simulink model "Quadcopter_Fix"  (R2021a)
settings: Solver=VariableStepAuto  StartTime=0.0  StopTime=50  RelTol=1e-3
values from neighbouring files (symbols this model uses):
  Ax = 0.0    (= 0)    [Quadcopter_Parameters.m]
  Ay = 0.0    (= 0)    [Quadcopter_Parameters.m]
  Az = 0.0    (= 0)    [Quadcopter_Parameters.m]
  b = 192.3208*10^(-7)    (= 1.923208e-05)    [Quadcopter_Parameters.m]
  d = 4.003*10^(-7)    (= 4.003e-07)    [Quadcopter_Parameters.m]
  g = 9.81    [Quadcopter_Parameters.m]
  Ixx = 15.67*10^(-3)    (= 0.01567)    [Quadcopter_Parameters.m]
  Iyy = 15.67*10^(-3)    (= 0.01567)    [Quadcopter_Parameters.m]
  Izz = 28.346*10^(-3)    (= 0.028346)    [Quadcopter_Parameters.m]
  Jr = 6.01*10^(-5)    (= 6.01e-05)    [Quadcopter_Parameters.m]
  l = 0.3    [Quadcopter_Parameters.m]
  m = weight/g    (= 0.815494393476)    [Quadcopter_Parameters.m]
undefined symbols (not defined in the file or in its folder): sigbuilder_block
libraries: pid_lib x6, vrlib x1
settings Model: Creator=Angga  LastModifiedBy=Angga
settings SolverCC: AlgebraicLoopSolver=TrustRegion
settings DataIOCC: ReturnWorkspaceOutputs=off
settings DebuggingCC: SFMachineParentedDataDiag=warning  ArithmeticOperatorsInVariantConditions=warning
settings SFSimCC: CustomCodeUndefinedFunction=UseInterfaceOnly

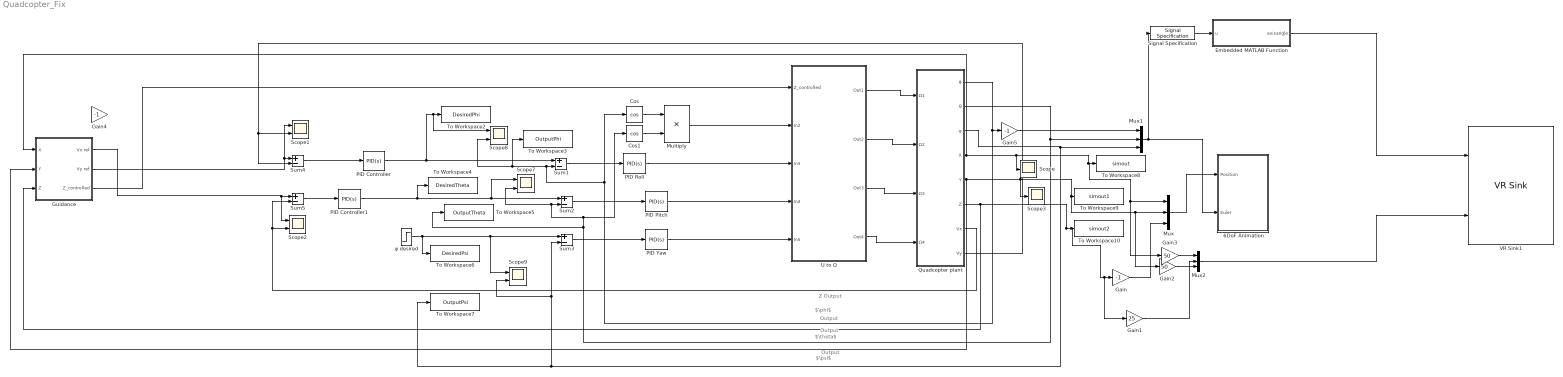
== system Quadcopter_Fix ==
  note: $\psi$
  note: $\theta$
  note: Output
  note: $\phi$
  note: Z Output
  note: Output
  note: Output
  "6DoF Animation " : Subsystem  mask{u1=[0 1 0 1 0 1], u2=0.03, u3=7, u4=[4000 0 -5000], u5=Fly alongside, u6=[-20 0 -7], u7=20, u8=off}
      mask prompts: u1 "Axes limits [xmin xmax ymin ymax zmin zmax]"; u2 "Time interval between updates:"; u3 "Size of craft displayed:"; u4 "Static object position [xp yp zp]"; u5 "Enter view:"; u6 "Position of camera [xc yc zc]"; u7 "View angle:"; u8 "Enable animation"
      mask init:
      | Config.axes = u1;
      | Config.update = u2;
      | Config.craft = u3;
      | Config.target = u4;
      | Config.camera_view = u5;
      | Config.camera_pos = u6;
      | Config.view = u7;
      | Config.Animenable = u8;
      | Config.Model = bdroot(gcb);
      mask TypeOptions u5: Fixed position | Cockpit | Fly alongside
      mask DialogControl DescGroupVar Prompt: 6DoF Animation
      mask Display:
      | port_label('input',1,'x_e','texmode','on');
      | port_label('input',2,'\phi \theta \psi','texmode','on');
      | [xp yp] = aeroimage('anim',gcbh);
      | patch(xp,yp)
  Cos : Trigonometry  Operator=cos
  Cos1 : Trigonometry  Operator=cos
  Embedded MATLAB Function : MATLAB Function  TreatAsAtomicUnit=on
  Gain : Gain  Gain=-1
  Gain1 : Gain  Gain=25
  Gain2 : Gain  Gain=50
  Gain3 : Gain  Gain=50
  Gain4 : Gain  Gain=-1
  Gain5 : Gain  Gain=-1
  Guidance : Subsystem
  Multiply : Product
  Mux : Mux  Inputs=3
  Mux1 : Mux  Inputs=3
  Mux2 : Mux  Inputs=3
  PID Controller : pid_lib/PID Controller  Controller=PID  Form=Parallel  TimeDomain=Continuous-time  UseExternalTs=off  SampleTime=-1  IntegratorMethod=Forward Euler  FilterMethod=Forward Euler  ControllerParametersSource=internal  P=-0.15  I=0  D=0  UseFilter=on  N=100  TunerSelectOption=Transfer Function Based (PID Tuner App)  InitialConditionSource=internal  InitialConditionForIntegrator=0  InitialConditionForFilter=0  DifferentiatorICPrevScaledInput=0  ExternalReset=none  TrackingMode=off  Kt=1  LimitOutput=off  SatLimitsSource=internal  UpperSaturationLimit=inf  LowerSaturationLimit=-inf  LinearizeAsGain=on  AntiWindupMode=none  Kb=1  POutMin=[]  POutMax=[]  IOutMin=[]  IOutMax=[]  DOutMin=[]  DOutMax=[]  NOutMin=[]  NOutMax=[]  SumOutMin=[]  SumOutMax=[]  SaturationOutMin=[]  SaturationOutMax=[]  PParamMin=[]  PParamMax=[]  IParamMin=[]  IParamMax=[]  DParamMin=[]  DParamMax=[]  NParamMin=[]  NParamMax=[]  KbParamMin=[]  KbParamMax=[]  KtParamMin=[]  KtParamMax=[]  KbOutMin=[]  KbOutMax=[]  KtOutMin=[]  KtOutMax=[]  IntegratorOutMin=[]  IntegratorOutMax=[]  FilterOutMin=[]  FilterOutMax=[]  SumI1OutMin=[]  SumI1OutMax=[]  SumI2OutMin=[]  SumI2OutMax=[]  SumI3OutMin=[]  SumI3OutMax=[]  SumI4OutMin=[]  SumI4OutMax=[]  SumDOutMin=[]  SumDOutMax=[]  DifferentiatorOutMin=[]  DifferentiatorOutMax=[]  FilterDiffOutCoefMin=[]  FilterDiffOutCoefMax=[]  ReciprocalOutMin=[]  ReciprocalOutMax=[]  SumDenOutMin=[]  SumDenOutMax=[]  SumNumOutMin=[]  SumNumOutMax=[]  DivideOutMin=[]  DivideOutMax=[]  UdiffTsProdOutMin=[]  UdiffTsProdOutMax=[]  NTsProdOutMin=[]  NTsProdOutMax=[]  UintegralTsProdOutMin=[]  UintegralTsProdOutMax=[]  UngainTsProdOutMin=[]  UngainTsProdOutMax=[]  IntegratorContinuousStateAttributes=''  IntegratorStateMustResolveToSignalObject=off  IntegratorRTWStateStorageClass=Auto  FilterContinuousStateAttributes=''  FilterStateMustResolveToSignalObject=off  FilterRTWStateStorageClass=Auto  ParallelPVariant=InternalParameters  IdealPVariant=Disabled  IVariant=InternalParameters  DVariant=InternalParameters  IntegratorVariant=Continuous  SatVariant=Disabled  AWVariant=Passthrough  PCopyVariant=Disabled  TRVariant=Disabled  FdbkBlocksVariant=Forward  IdealPFdbkVariant=Disabled  SatFdbkVariant=Disabled  DerivativeFilterVariant=ContFilter  NVariant=InternalParameters  NCopyVariant=Disabled  FilterICVariant=InternalICsFilter  IntegratorICVariant=InternalICs  ExternalResetVariant=Disabled  TRSumVariant=Passthrough  SumFdbkVariant=Disabled  SumVariant=Sum_PID  TsampFilterVariant=InternalTs  TsampNgainVariant=Passthrough  TsampIntegralVariant=Passthrough  ExternalSaturationOutDataTypeStr=Inherit: Same as second input
  PID Controller1 : pid_lib/PID Controller  Controller=PID  Form=Parallel  TimeDomain=Continuous-time  UseExternalTs=off  SampleTime=-1  IntegratorMethod=Forward Euler  FilterMethod=Forward Euler  ControllerParametersSource=internal  P=-0.2  I=0  D=0  UseFilter=on  N=100  TunerSelectOption=Transfer Function Based (PID Tuner App)  InitialConditionSource=internal  InitialConditionForIntegrator=0  InitialConditionForFilter=0  DifferentiatorICPrevScaledInput=0  ExternalReset=none  TrackingMode=off  Kt=1  LimitOutput=off  SatLimitsSource=internal  UpperSaturationLimit=inf  LowerSaturationLimit=-inf  LinearizeAsGain=on  AntiWindupMode=none  Kb=1  POutMin=[]  POutMax=[]  IOutMin=[]  IOutMax=[]  DOutMin=[]  DOutMax=[]  NOutMin=[]  NOutMax=[]  SumOutMin=[]  SumOutMax=[]  SaturationOutMin=[]  SaturationOutMax=[]  PParamMin=[]  PParamMax=[]  IParamMin=[]  IParamMax=[]  DParamMin=[]  DParamMax=[]  NParamMin=[]  NParamMax=[]  KbParamMin=[]  KbParamMax=[]  KtParamMin=[]  KtParamMax=[]  KbOutMin=[]  KbOutMax=[]  KtOutMin=[]  KtOutMax=[]  IntegratorOutMin=[]  IntegratorOutMax=[]  FilterOutMin=[]  FilterOutMax=[]  SumI1OutMin=[]  SumI1OutMax=[]  SumI2OutMin=[]  SumI2OutMax=[]  SumI3OutMin=[]  SumI3OutMax=[]  SumI4OutMin=[]  SumI4OutMax=[]  SumDOutMin=[]  SumDOutMax=[]  DifferentiatorOutMin=[]  DifferentiatorOutMax=[]  FilterDiffOutCoefMin=[]  FilterDiffOutCoefMax=[]  ReciprocalOutMin=[]  ReciprocalOutMax=[]  SumDenOutMin=[]  SumDenOutMax=[]  SumNumOutMin=[]  SumNumOutMax=[]  DivideOutMin=[]  DivideOutMax=[]  UdiffTsProdOutMin=[]  UdiffTsProdOutMax=[]  NTsProdOutMin=[]  NTsProdOutMax=[]  UintegralTsProdOutMin=[]  UintegralTsProdOutMax=[]  UngainTsProdOutMin=[]  UngainTsProdOutMax=[]  IntegratorContinuousStateAttributes=''  IntegratorStateMustResolveToSignalObject=off  IntegratorRTWStateStorageClass=Auto  FilterContinuousStateAttributes=''  FilterStateMustResolveToSignalObject=off  FilterRTWStateStorageClass=Auto  ParallelPVariant=InternalParameters  IdealPVariant=Disabled  IVariant=InternalParameters  DVariant=InternalParameters  IntegratorVariant=Continuous  SatVariant=Disabled  AWVariant=Passthrough  PCopyVariant=Disabled  TRVariant=Disabled  FdbkBlocksVariant=Forward  IdealPFdbkVariant=Disabled  SatFdbkVariant=Disabled  DerivativeFilterVariant=ContFilter  NVariant=InternalParameters  NCopyVariant=Disabled  FilterICVariant=InternalICsFilter  IntegratorICVariant=InternalICs  ExternalResetVariant=Disabled  TRSumVariant=Passthrough  SumFdbkVariant=Disabled  SumVariant=Sum_PID  TsampFilterVariant=InternalTs  TsampNgainVariant=Passthrough  TsampIntegralVariant=Passthrough  ExternalSaturationOutDataTypeStr=Inherit: Same as second input
  PID Pitch : pid_lib/PID Controller  Controller=PID  Form=Parallel  TimeDomain=Continuous-time  UseExternalTs=off  SampleTime=-1  IntegratorMethod=Forward Euler  FilterMethod=Forward Euler  ControllerParametersSource=internal  P=0.05  I=0  D=0.05  UseFilter=on  N=100  TunerSelectOption=Transfer Function Based (PID Tuner App)  InitialConditionSource=internal  InitialConditionForIntegrator=0  InitialConditionForFilter=0  DifferentiatorICPrevScaledInput=0  ExternalReset=none  TrackingMode=off  Kt=1  LimitOutput=off  SatLimitsSource=internal  UpperSaturationLimit=inf  LowerSaturationLimit=-inf  LinearizeAsGain=on  AntiWindupMode=none  Kb=1  POutMin=[]  POutMax=[]  IOutMin=[]  IOutMax=[]  DOutMin=[]  DOutMax=[]  NOutMin=[]  NOutMax=[]  SumOutMin=[]  SumOutMax=[]  SaturationOutMin=[]  SaturationOutMax=[]  PParamMin=[]  PParamMax=[]  IParamMin=[]  IParamMax=[]  DParamMin=[]  DParamMax=[]  NParamMin=[]  NParamMax=[]  KbParamMin=[]  KbParamMax=[]  KtParamMin=[]  KtParamMax=[]  KbOutMin=[]  KbOutMax=[]  KtOutMin=[]  KtOutMax=[]  IntegratorOutMin=[]  IntegratorOutMax=[]  FilterOutMin=[]  FilterOutMax=[]  SumI1OutMin=[]  SumI1OutMax=[]  SumI2OutMin=[]  SumI2OutMax=[]  SumI3OutMin=[]  SumI3OutMax=[]  SumI4OutMin=[]  SumI4OutMax=[]  SumDOutMin=[]  SumDOutMax=[]  DifferentiatorOutMin=[]  DifferentiatorOutMax=[]  FilterDiffOutCoefMin=[]  FilterDiffOutCoefMax=[]  ReciprocalOutMin=[]  ReciprocalOutMax=[]  SumDenOutMin=[]  SumDenOutMax=[]  SumNumOutMin=[]  SumNumOutMax=[]  DivideOutMin=[]  DivideOutMax=[]  UdiffTsProdOutMin=[]  UdiffTsProdOutMax=[]  NTsProdOutMin=[]  NTsProdOutMax=[]  UintegralTsProdOutMin=[]  UintegralTsProdOutMax=[]  UngainTsProdOutMin=[]  UngainTsProdOutMax=[]  IntegratorContinuousStateAttributes=''  IntegratorStateMustResolveToSignalObject=off  IntegratorRTWStateStorageClass=Auto  FilterContinuousStateAttributes=''  FilterStateMustResolveToSignalObject=off  FilterRTWStateStorageClass=Auto  ParallelPVariant=InternalParameters  IdealPVariant=Disabled  IVariant=InternalParameters  DVariant=InternalParameters  IntegratorVariant=Continuous  SatVariant=Disabled  AWVariant=Passthrough  PCopyVariant=Disabled  TRVariant=Disabled  FdbkBlocksVariant=Forward  IdealPFdbkVariant=Disabled  SatFdbkVariant=Disabled  DerivativeFilterVariant=ContFilter  NVariant=InternalParameters  NCopyVariant=Disabled  FilterICVariant=InternalICsFilter  IntegratorICVariant=InternalICs  ExternalResetVariant=Disabled  TRSumVariant=Passthrough  SumFdbkVariant=Disabled  SumVariant=Sum_PID  TsampFilterVariant=InternalTs  TsampNgainVariant=Passthrough  TsampIntegralVariant=Passthrough  ExternalSaturationOutDataTypeStr=Inherit: Same as second input
  PID Roll : pid_lib/PID Controller  Controller=PID  Form=Parallel  TimeDomain=Continuous-time  UseExternalTs=off  SampleTime=-1  IntegratorMethod=Forward Euler  FilterMethod=Forward Euler  ControllerParametersSource=internal  P=0.05  I=0  D=0.05  UseFilter=on  N=100  TunerSelectOption=Transfer Function Based (PID Tuner App)  InitialConditionSource=internal  InitialConditionForIntegrator=0  InitialConditionForFilter=0  DifferentiatorICPrevScaledInput=0  ExternalReset=none  TrackingMode=off  Kt=1  LimitOutput=off  SatLimitsSource=internal  UpperSaturationLimit=inf  LowerSaturationLimit=-inf  LinearizeAsGain=on  AntiWindupMode=none  Kb=1  POutMin=[]  POutMax=[]  IOutMin=[]  IOutMax=[]  DOutMin=[]  DOutMax=[]  NOutMin=[]  NOutMax=[]  SumOutMin=[]  SumOutMax=[]  SaturationOutMin=[]  SaturationOutMax=[]  PParamMin=[]  PParamMax=[]  IParamMin=[]  IParamMax=[]  DParamMin=[]  DParamMax=[]  NParamMin=[]  NParamMax=[]  KbParamMin=[]  KbParamMax=[]  KtParamMin=[]  KtParamMax=[]  KbOutMin=[]  KbOutMax=[]  KtOutMin=[]  KtOutMax=[]  IntegratorOutMin=[]  IntegratorOutMax=[]  FilterOutMin=[]  FilterOutMax=[]  SumI1OutMin=[]  SumI1OutMax=[]  SumI2OutMin=[]  SumI2OutMax=[]  SumI3OutMin=[]  SumI3OutMax=[]  SumI4OutMin=[]  SumI4OutMax=[]  SumDOutMin=[]  SumDOutMax=[]  DifferentiatorOutMin=[]  DifferentiatorOutMax=[]  FilterDiffOutCoefMin=[]  FilterDiffOutCoefMax=[]  ReciprocalOutMin=[]  ReciprocalOutMax=[]  SumDenOutMin=[]  SumDenOutMax=[]  SumNumOutMin=[]  SumNumOutMax=[]  DivideOutMin=[]  DivideOutMax=[]  UdiffTsProdOutMin=[]  UdiffTsProdOutMax=[]  NTsProdOutMin=[]  NTsProdOutMax=[]  UintegralTsProdOutMin=[]  UintegralTsProdOutMax=[]  UngainTsProdOutMin=[]  UngainTsProdOutMax=[]  IntegratorContinuousStateAttributes=''  IntegratorStateMustResolveToSignalObject=off  IntegratorRTWStateStorageClass=Auto  FilterContinuousStateAttributes=''  FilterStateMustResolveToSignalObject=off  FilterRTWStateStorageClass=Auto  ParallelPVariant=InternalParameters  IdealPVariant=Disabled  IVariant=InternalParameters  DVariant=InternalParameters  IntegratorVariant=Continuous  SatVariant=Disabled  AWVariant=Passthrough  PCopyVariant=Disabled  TRVariant=Disabled  FdbkBlocksVariant=Forward  IdealPFdbkVariant=Disabled  SatFdbkVariant=Disabled  DerivativeFilterVariant=ContFilter  NVariant=InternalParameters  NCopyVariant=Disabled  FilterICVariant=InternalICsFilter  IntegratorICVariant=InternalICs  ExternalResetVariant=Disabled  TRSumVariant=Passthrough  SumFdbkVariant=Disabled  SumVariant=Sum_PID  TsampFilterVariant=InternalTs  TsampNgainVariant=Passthrough  TsampIntegralVariant=Passthrough  ExternalSaturationOutDataTypeStr=Inherit: Same as second input
  PID Yaw : pid_lib/PID Controller  Controller=PID  Form=Parallel  TimeDomain=Continuous-time  UseExternalTs=off  SampleTime=-1  IntegratorMethod=Forward Euler  FilterMethod=Forward Euler  ControllerParametersSource=internal  P=0.05  I=0  D=0.05  UseFilter=on  N=100  TunerSelectOption=Transfer Function Based (PID Tuner App)  InitialConditionSource=internal  InitialConditionForIntegrator=0  InitialConditionForFilter=0  DifferentiatorICPrevScaledInput=0  ExternalReset=none  TrackingMode=off  Kt=1  LimitOutput=off  SatLimitsSource=internal  UpperSaturationLimit=inf  LowerSaturationLimit=-inf  LinearizeAsGain=on  AntiWindupMode=none  Kb=1  POutMin=[]  POutMax=[]  IOutMin=[]  IOutMax=[]  DOutMin=[]  DOutMax=[]  NOutMin=[]  NOutMax=[]  SumOutMin=[]  SumOutMax=[]  SaturationOutMin=[]  SaturationOutMax=[]  PParamMin=[]  PParamMax=[]  IParamMin=[]  IParamMax=[]  DParamMin=[]  DParamMax=[]  NParamMin=[]  NParamMax=[]  KbParamMin=[]  KbParamMax=[]  KtParamMin=[]  KtParamMax=[]  KbOutMin=[]  KbOutMax=[]  KtOutMin=[]  KtOutMax=[]  IntegratorOutMin=[]  IntegratorOutMax=[]  FilterOutMin=[]  FilterOutMax=[]  SumI1OutMin=[]  SumI1OutMax=[]  SumI2OutMin=[]  SumI2OutMax=[]  SumI3OutMin=[]  SumI3OutMax=[]  SumI4OutMin=[]  SumI4OutMax=[]  SumDOutMin=[]  SumDOutMax=[]  DifferentiatorOutMin=[]  DifferentiatorOutMax=[]  FilterDiffOutCoefMin=[]  FilterDiffOutCoefMax=[]  ReciprocalOutMin=[]  ReciprocalOutMax=[]  SumDenOutMin=[]  SumDenOutMax=[]  SumNumOutMin=[]  SumNumOutMax=[]  DivideOutMin=[]  DivideOutMax=[]  UdiffTsProdOutMin=[]  UdiffTsProdOutMax=[]  NTsProdOutMin=[]  NTsProdOutMax=[]  UintegralTsProdOutMin=[]  UintegralTsProdOutMax=[]  UngainTsProdOutMin=[]  UngainTsProdOutMax=[]  IntegratorContinuousStateAttributes=''  IntegratorStateMustResolveToSignalObject=off  IntegratorRTWStateStorageClass=Auto  FilterContinuousStateAttributes=''  FilterStateMustResolveToSignalObject=off  FilterRTWStateStorageClass=Auto  ParallelPVariant=InternalParameters  IdealPVariant=Disabled  IVariant=InternalParameters  DVariant=InternalParameters  IntegratorVariant=Continuous  SatVariant=Disabled  AWVariant=Passthrough  PCopyVariant=Disabled  TRVariant=Disabled  FdbkBlocksVariant=Forward  IdealPFdbkVariant=Disabled  SatFdbkVariant=Disabled  DerivativeFilterVariant=ContFilter  NVariant=InternalParameters  NCopyVariant=Disabled  FilterICVariant=InternalICsFilter  IntegratorICVariant=InternalICs  ExternalResetVariant=Disabled  TRSumVariant=Passthrough  SumFdbkVariant=Disabled  SumVariant=Sum_PID  TsampFilterVariant=InternalTs  TsampNgainVariant=Passthrough  TsampIntegralVariant=Passthrough  ExternalSaturationOutDataTypeStr=Inherit: Same as second input
  Quadcopter plant : Subsystem
  Scope : Scope
  Scope{1..2,7..9} (5 alike) : Scope  NumInputPorts=2
  Scope3 : Scope
  Signal Specification : SignalSpecification  Dimensions=3
  Sum{1..5} (5 alike) : Sum  Inputs=+-
  To Workspace10 : ToWorkspace  VariableName=simout2  SampleTime=-1
  To Workspace2 : ToWorkspace  VariableName=DesiredPhi  SampleTime=-1
  To Workspace3 : ToWorkspace  VariableName=OutputPhi  SampleTime=-1
  To Workspace4 : ToWorkspace  VariableName=DesiredTheta  SampleTime=-1
  To Workspace5 : ToWorkspace  VariableName=OutputTheta  SampleTime=-1
  To Workspace6 : ToWorkspace  VariableName=DesiredPsi  SampleTime=-1
  To Workspace7 : ToWorkspace  VariableName=OutputPsi  SampleTime=-1
  To Workspace8 : ToWorkspace  VariableName=simout  SampleTime=-1
  To Workspace9 : ToWorkspace  VariableName=simout1  SampleTime=-1
  U to Ω : Subsystem
  VR Sink1 : vrlib/VR Sink  InstantiateOnLoad=on  SampleTime=0.05  ViewEnable=on  RemoteChange=off  RemoteView=on  FieldsWritten=STLB_Transform.rotation.4.1.1.double#STLB_Transform.translation.3.1.1.double  WorldFileName=Quadcopter.x3d  AutoView=on  VideoDimensions=[]  AllowVariableSize=off
  ψ desired : Step  After=0  SampleTime=0
  wires:
  Quadcopter plant/3(ψ) -> Sum3/2, Scope9/2, To Workspace7/1, Mux1/3
  Quadcopter plant/4(X) -> Guidance/1(X), Scope/1, Gain3/1, Mux/1, To Workspace8/1
  Quadcopter plant/1(ϕ) -> To Workspace3/1, Scope8/2, Sum1/2, Cos/1, Gain5/1
  Quadcopter plant/2(θ) -> Cos1/1, Scope7/2, Sum2/2, To Workspace5/1, Mux1/2
  Quadcopter plant/6(Z) -> Guidance/3(Z), Gain1/1, Gain/1, To Workspace10/1
  Cos/1 -> Multiply/1
  Cos1/1 -> Multiply/2
  Sum1/1 -> PID Roll/1
  Sum2/1 -> PID Pitch/1
  ψ desired/1 -> To Workspace6/1, Scope9/1, Sum3/1
  Sum3/1 -> PID Yaw/1
  Mux/1 -> "6DoF Animation "/1(Position)
  Mux1/1 -> Signal Specification/1, "6DoF Animation "/2(Euler)
  Gain/1 -> Mux/3
  Multiply/1 -> U to Ω/2(In2)
  PID Roll/1 -> U to Ω/3(In3)
  PID Pitch/1 -> U to Ω/4(In4)
  PID Yaw/1 -> U to Ω/5(In5)
  U to Ω/1(Out1) -> Quadcopter plant/1(Ω1)
  U to Ω/2(Out2) -> Quadcopter plant/2(Ω2)
  U to Ω/3(Out3) -> Quadcopter plant/3(Ω3)
  U to Ω/4(Out4) -> Quadcopter plant/4(Ω4)
  Signal Specification/1 -> Embedded MATLAB Function/1(u)
  Embedded MATLAB Function/1(axisangle) -> VR Sink1/1
  Mux2/1 -> VR Sink1/2
  Gain1/1 -> Mux2/2
  PID Controller/1 -> Sum1/1, Scope8/1, To Workspace2/1
  PID Controller1/1 -> To Workspace4/1, Sum2/1, Scope7/1
  Quadcopter plant/8(Vy) -> Scope1/2, Sum4/2
  Sum4/1 -> PID Controller/1
  Quadcopter plant/7(Vx) -> Sum5/2, Scope2/2
  Sum5/1 -> PID Controller1/1
  Guidance/3(Z_controlled) -> U to Ω/1(Z_controlled)
  Guidance/2(Vy ref) -> Scope1/1, Sum4/1
  Guidance/1(Vx ref) -> Scope2/1, Sum5/1
  Gain2/1 -> Mux2/3
  Gain3/1 -> Mux2/1
  Quadcopter plant/5(Y) -> Scope3/1, Gain2/1, Mux/2, To Workspace9/1, Guidance/2(Y)
  Gain5/1 -> Mux1/1

== system Quadcopter_Fix/6DoF Animation  ==
  Position : Inport
  Euler : Inport  Port=2
  Animation S-Function : S-Function  FunctionName=sixdofanim  Parameters=Config  SFunctionDeploymentMode=off  EnableBusSupport=off
  Mux3 : Mux  Inputs=2
  wires:
  Mux3/1 -> Animation S-Function/1
  Position/1 -> Mux3/1
  Euler/1 -> Mux3/2

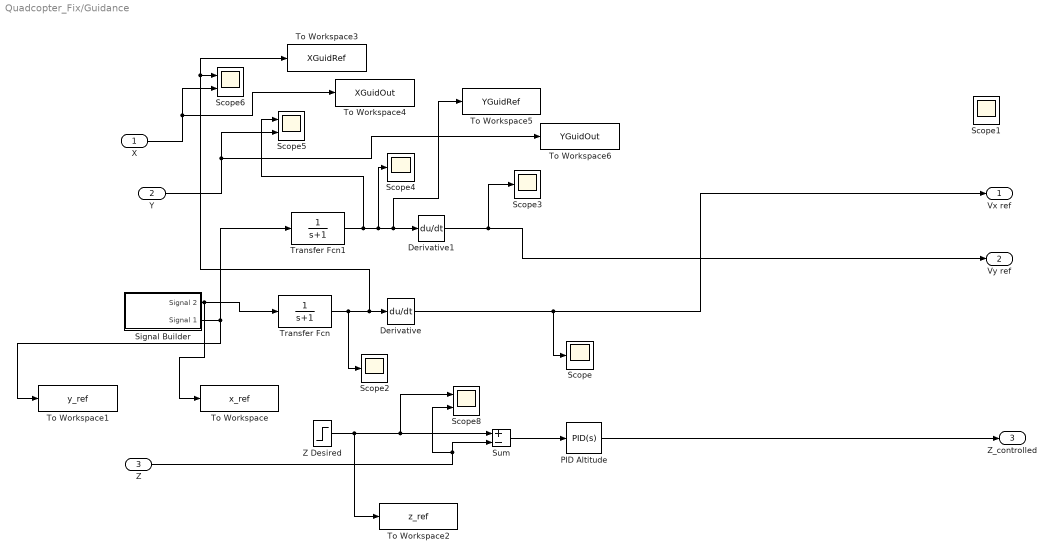
== system Quadcopter_Fix/Guidance ==
  X : Inport
  Y : Inport  Port=2
  Z : Inport  Port=3
  Derivative : Derivative
  Derivative1 : Derivative
  PID Altitude : pid_lib/PID Controller  Controller=PID  Form=Parallel  TimeDomain=Continuous-time  UseExternalTs=off  SampleTime=-1  IntegratorMethod=Forward Euler  FilterMethod=Forward Euler  ControllerParametersSource=internal  P=6  I=3  D=3  UseFilter=on  N=100  TunerSelectOption=Transfer Function Based (PID Tuner App)  InitialConditionSource=internal  InitialConditionForIntegrator=0  InitialConditionForFilter=0  DifferentiatorICPrevScaledInput=0  ExternalReset=none  TrackingMode=off  Kt=1  LimitOutput=off  SatLimitsSource=internal  UpperSaturationLimit=inf  LowerSaturationLimit=-inf  LinearizeAsGain=on  AntiWindupMode=none  Kb=1  POutMin=[]  POutMax=[]  IOutMin=[]  IOutMax=[]  DOutMin=[]  DOutMax=[]  NOutMin=[]  NOutMax=[]  SumOutMin=[]  SumOutMax=[]  SaturationOutMin=[]  SaturationOutMax=[]  PParamMin=[]  PParamMax=[]  IParamMin=[]  IParamMax=[]  DParamMin=[]  DParamMax=[]  NParamMin=[]  NParamMax=[]  KbParamMin=[]  KbParamMax=[]  KtParamMin=[]  KtParamMax=[]  KbOutMin=[]  KbOutMax=[]  KtOutMin=[]  KtOutMax=[]  IntegratorOutMin=[]  IntegratorOutMax=[]  FilterOutMin=[]  FilterOutMax=[]  SumI1OutMin=[]  SumI1OutMax=[]  SumI2OutMin=[]  SumI2OutMax=[]  SumI3OutMin=[]  SumI3OutMax=[]  SumI4OutMin=[]  SumI4OutMax=[]  SumDOutMin=[]  SumDOutMax=[]  DifferentiatorOutMin=[]  DifferentiatorOutMax=[]  FilterDiffOutCoefMin=[]  FilterDiffOutCoefMax=[]  ReciprocalOutMin=[]  ReciprocalOutMax=[]  SumDenOutMin=[]  SumDenOutMax=[]  SumNumOutMin=[]  SumNumOutMax=[]  DivideOutMin=[]  DivideOutMax=[]  UdiffTsProdOutMin=[]  UdiffTsProdOutMax=[]  NTsProdOutMin=[]  NTsProdOutMax=[]  UintegralTsProdOutMin=[]  UintegralTsProdOutMax=[]  UngainTsProdOutMin=[]  UngainTsProdOutMax=[]  IntegratorContinuousStateAttributes=''  IntegratorStateMustResolveToSignalObject=off  IntegratorRTWStateStorageClass=Auto  FilterContinuousStateAttributes=''  FilterStateMustResolveToSignalObject=off  FilterRTWStateStorageClass=Auto  ParallelPVariant=InternalParameters  IdealPVariant=Disabled  IVariant=InternalParameters  DVariant=InternalParameters  IntegratorVariant=Continuous  SatVariant=Disabled  AWVariant=Passthrough  PCopyVariant=Disabled  TRVariant=Disabled  FdbkBlocksVariant=Forward  IdealPFdbkVariant=Disabled  SatFdbkVariant=Disabled  DerivativeFilterVariant=ContFilter  NVariant=InternalParameters  NCopyVariant=Disabled  FilterICVariant=InternalICsFilter  IntegratorICVariant=InternalICs  ExternalResetVariant=Disabled  TRSumVariant=Passthrough  SumFdbkVariant=Disabled  SumVariant=Sum_PID  TsampFilterVariant=InternalTs  TsampNgainVariant=Passthrough  TsampIntegralVariant=Passthrough  ExternalSaturationOutDataTypeStr=Inherit: Same as second input
  Scope{,1..4} (5 alike) : Scope
  Scope5 : Scope  NumInputPorts=2
  Scope6 : Scope  NumInputPorts=2
  Scope8 : Scope  NumInputPorts=2
  Signal Builder : Subsystem  Tag=STV Subsys  LoadFcn=sigbuilder_block('load');  StartFcn=sigbuilder_block('start');  StopFcn=sigbuilder_block('stop');  ClipboardFcn=sigbuilder_block('clipboard');  mask(Sigbuilder block){tuvar=[0:10]}
      mask help: Simulink:masks:SigbuilderBlock_MD
      mask init:
      | if ~strcmp(get_param(bdroot(gcbh),'SimulationStatus'),'stopped') tuvar = sigbuilder_block('maskInit'); end
      settings: CopyFcn=sigbuilder_block('copy');  DeleteFcn=sigbuilder_block('delete');  ModelCloseFcn=sigbuilder_block('modelClose');  PreSaveFcn=sigbuilder_block('preSave');  PauseFcn=sigbuilder_block('pause');  ContinueFcn=sigbuilder_block('continue');  NameChangeFcn=sigbuilder_block('namechange');  OpenFcn=sigbuilder_block('open',[5.5 -8 949 380.5 ]);  CloseFcn=sigbuilder_block('close');
      mask Display: plot(0, 0, 100, 100,[2, 2, 32, 32, 2], [68, 8, 8, 68, 68],[32, 2], [38, 38], [32, 19, 2],[53, 60, 44], [32, 17, 17, 2],[16, 16, 31, 31]);txt = getActiveGroup(gcbh);text(2, 100, txt,'verticalAlignment', 'top');
  Sum : Sum  Inputs=+-
  To Workspace : ToWorkspace  VariableName=x_ref  SampleTime=-1
  To Workspace1 : ToWorkspace  VariableName=y_ref  SampleTime=-1
  To Workspace2 : ToWorkspace  VariableName=z_ref  SampleTime=-1
  To Workspace3 : ToWorkspace  VariableName=XGuidRef  SampleTime=-1
  To Workspace4 : ToWorkspace  VariableName=XGuidOut  SampleTime=-1
  To Workspace5 : ToWorkspace  VariableName=YGuidRef  SampleTime=-1
  To Workspace6 : ToWorkspace  VariableName=YGuidOut  SampleTime=-1
  Transfer Fcn : TransferFcn  Denominator=[1 1]
  Transfer Fcn1 : TransferFcn  Denominator=[1 1]
  Z Desired : Step  After=5  SampleTime=0
  Vx ref : Outport
  Vy ref : Outport  Port=2
  Z_controlled : Outport  Port=3
  wires:
  Sum/1 -> PID Altitude/1
  Z Desired/1 -> To Workspace2/1, Scope8/1, Sum/1
  Z/1 -> Scope8/2, Sum/2
  PID Altitude/1 -> Z_controlled/1
  Signal Builder/1(Signal 2) -> To Workspace/1, Transfer Fcn/1
  Transfer Fcn/1 -> Scope2/1, To Workspace3/1, Scope6/1, Derivative/1
  Derivative/1 -> Scope/1, Vx ref/1
  Signal Builder/2(Signal 1) -> To Workspace1/1, Transfer Fcn1/1
  Transfer Fcn1/1 -> Scope5/1, Scope4/1, To Workspace5/1, Derivative1/1
  Derivative1/1 -> Scope3/1, Vy ref/1
  Y/1 -> To Workspace6/1, Scope5/2
  X/1 -> To Workspace4/1, Scope6/2

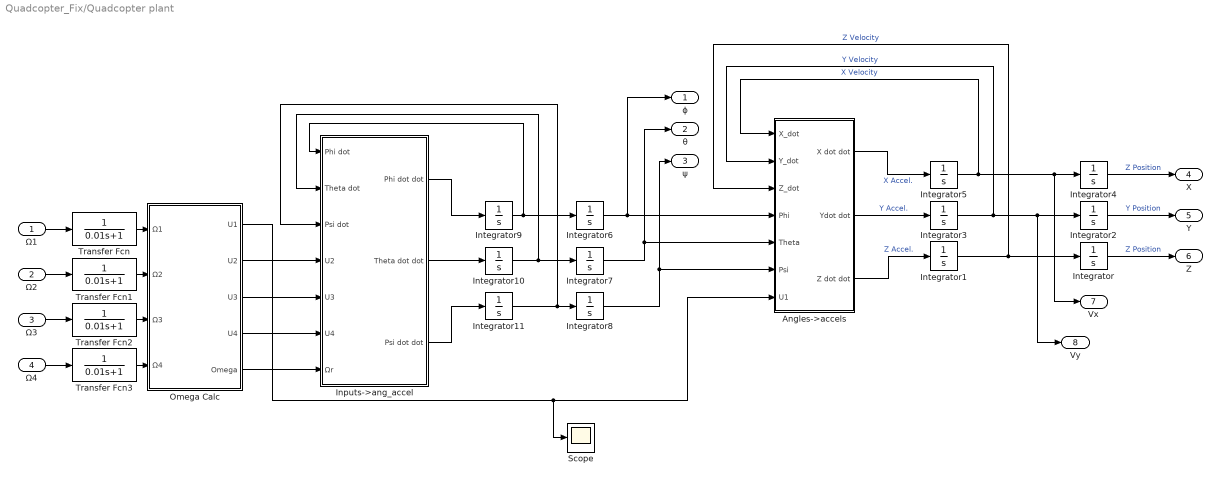
== system Quadcopter_Fix/Quadcopter plant ==
  Ω1 : Inport
  Ω2 : Inport  Port=2
  Ω3 : Inport  Port=3
  Ω4 : Inport  Port=4
  Angles->accels : Subsystem
  Inputs->ang_accel : Subsystem
  Integrator : Integrator  LimitOutput=on  LowerSaturationLimit=0
  Integrator{1..5,8..9} (7 alike) : Integrator
  Integrator10 : Integrator  UpperSaturationLimit=10000  LowerSaturationLimit=-10000
  Integrator11 : Integrator  UpperSaturationLimit=10000  LowerSaturationLimit=-10000
  Integrator6 : Integrator  WrapState=on  WrappedStateUpperValue=pi/2  WrappedStateLowerValue=-pi/2
  Integrator7 : Integrator  WrapState=on  WrappedStateUpperValue=pi/3  WrappedStateLowerValue=-pi/3
  Omega Calc : Subsystem
  Scope : Scope
  Transfer Fcn{,1..3} (4 alike) : TransferFcn  Denominator=[0.01 1]
  ϕ : Outport  VectorParamsAs1DForOutWhenUnconnected=off
  θ : Outport  Port=2  VectorParamsAs1DForOutWhenUnconnected=off
  ψ : Outport  Port=3  VectorParamsAs1DForOutWhenUnconnected=off
  X : Outport  Port=4  VectorParamsAs1DForOutWhenUnconnected=off
  Y : Outport  Port=5  VectorParamsAs1DForOutWhenUnconnected=off
  Z : Outport  Port=6  VectorParamsAs1DForOutWhenUnconnected=off
  Vx : Outport  Port=7  VectorParamsAs1DForOutWhenUnconnected=off
  Vy : Outport  Port=8  VectorParamsAs1DForOutWhenUnconnected=off
  wires:
  Integrator1/1 -> Angles->accels/3(Z_dot), Integrator/1  "Z Velocity"
  Integrator2/1 -> Y/1  "Y Position"
  Integrator3/1 -> Angles->accels/2(Y_dot), Vy/1, Integrator2/1  "Y Velocity"
  Angles->accels/2(Ydot dot) -> Integrator3/1  "Y Accel."
  Angles->accels/3(Z dot dot) -> Integrator1/1  "Z Accel."
  Integrator8/1 -> Angles->accels/6(Psi), ψ/1
  Integrator7/1 -> Angles->accels/5(Theta), θ/1
  Integrator6/1 -> Angles->accels/4(Phi), ϕ/1
  Integrator11/1 -> Inputs->ang_accel/3(Psi dot), Integrator8/1
  Integrator10/1 -> Inputs->ang_accel/2(Theta dot), Integrator7/1
  Integrator9/1 -> Inputs->ang_accel/1(Phi dot), Integrator6/1
  Inputs->ang_accel/2(Theta dot dot) -> Integrator10/1
  Inputs->ang_accel/1(Phi dot dot) -> Integrator9/1
  Inputs->ang_accel/3(Psi dot dot) -> Integrator11/1
  Omega Calc/5(Omega) -> Inputs->ang_accel/7(Ωr)
  Omega Calc/4(U4) -> Inputs->ang_accel/6(U4)
  Omega Calc/3(U3) -> Inputs->ang_accel/5(U3)
  Omega Calc/2(U2) -> Inputs->ang_accel/4(U2)
  Omega Calc/1(U1) -> Scope/1, Angles->accels/7(U1)
  Integrator5/1 -> Angles->accels/1(X_dot), Vx/1, Integrator4/1  "X Velocity"
  Angles->accels/1(X dot dot) -> Integrator5/1  "X Accel."
  Integrator4/1 -> X/1  "Z Position"
  Integrator/1 -> Z/1  "Z Position"
  Transfer Fcn/1 -> Omega Calc/1(Ω1)
  Ω1/1 -> Transfer Fcn/1
  Transfer Fcn1/1 -> Omega Calc/2(Ω2)
  Ω2/1 -> Transfer Fcn1/1
  Transfer Fcn3/1 -> Omega Calc/4(Ω4)
  Ω4/1 -> Transfer Fcn3/1
  Ω3/1 -> Transfer Fcn2/1
  Transfer Fcn2/1 -> Omega Calc/3(Ω3)

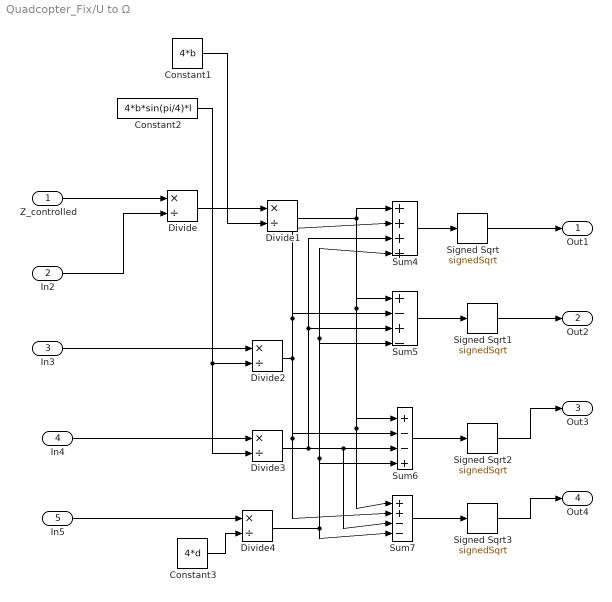
== system Quadcopter_Fix/U to Ω ==
  Z_controlled : Inport
  In2 : Inport  Port=2
  In3 : Inport  Port=3
  In4 : Inport  Port=4
  In5 : Inport  Port=5
  Constant1 : Constant  Value=4*b
  Constant2 : Constant  Value=4*b*sin(pi/4)*l
  Constant3 : Constant  Value=4*d
  Divide{,1..4} (5 alike) : Product  Inputs=*/
  Signed Sqrt{,1..3} (4 alike) : Sqrt  Operator=signedSqrt  SaturateOnIntegerOverflow=on
  Sum4 : Sum  Inputs=|++++
  Sum5 : Sum  Inputs=|+-+-
  Sum6 : Sum  Inputs=|+--+
  Sum7 : Sum  Inputs=|++--
  Out1 : Outport
  Out2 : Outport  Port=2
  Out3 : Outport  Port=3
  Out4 : Outport  Port=4
  wires:
  Constant2/1 -> Divide2/2, Divide3/2
  Divide1/1 -> Sum7/1, Sum6/1, Sum5/1, Sum4/1
  Sum6/1 -> Signed Sqrt2/1
  Sum7/1 -> Signed Sqrt3/1
  Signed Sqrt/1 -> Out1/1
  Constant1/1 -> Divide1/2
  Divide2/1 -> Sum7/2, Sum6/2, Sum4/2, Sum5/2
  Constant3/1 -> Divide4/2
  Sum4/1 -> Signed Sqrt/1
  Divide/1 -> Divide1/1
  In2/1 -> Divide/2
  Divide3/1 -> Sum4/3, Sum5/3, Sum7/3, Sum6/3
  In3/1 -> Divide2/1
  Divide4/1 -> Sum7/4, Sum6/4, Sum4/4, Sum5/4
  In5/1 -> Divide4/1
  Sum5/1 -> Signed Sqrt1/1
  In4/1 -> Divide3/1
  Z_controlled/1 -> Divide/1
  Signed Sqrt1/1 -> Out2/1
  Signed Sqrt3/1 -> Out4/1
  Signed Sqrt2/1 -> Out3/1

== system Quadcopter_Fix/Guidance/Signal Builder ==
  Demux : Demux  Tag=STV Demux  Outputs=2
      settings: DisplayOption=none
  FromWs : FromWorkspace  Tag=STV FromWs  VariableName=tuvar
      SigBuilderData=|
      | common.afterFinalStr = 'Extrapolate'
      | common.sampleTime = 0
      | dataSet.timeRange = [0 50]
      | dataSet.name = 'Group 1'
      | sbobj.Groups.Name = 'Group 1'
      | sbobj.Groups.Signals(1).Name = 'Signal 2'
      | sbobj.Groups.Signals(1).XData = [0 10.1 10.1 20 30 30 40 50]
      | sbobj.Groups.Signals(1).YData = [0 0 5.05 5.05 5 0 0 -0.02]
      | sbobj.Groups.Signals(2).Name = 'Signal 1'
      | sbobj.Groups.Signals(2).XData = [0 20 20 30 40 40 50]
      | sbobj.Groups.Signals(2).YData = [0 0 5 5 5 0 0]
      | sbobj.Groups.TimeRange = [0 50]
  Signal 2 : Outport  Tag=STV Outport
  Signal 1 : Outport  Tag=STV Outport  Port=2
  wires:
  FromWs/1 -> Demux/1
  Demux/1 -> Signal 2/1
  Demux/2 -> Signal 1/1

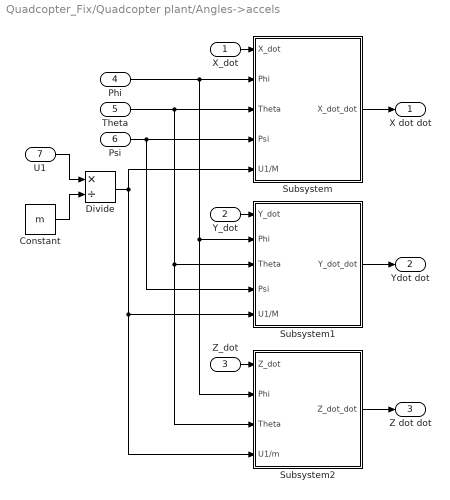
== system Quadcopter_Fix/Quadcopter plant/Angles->accels ==
  X_dot : Inport
  Y_dot : Inport  Port=2
  Z_dot : Inport  Port=3
  Phi : Inport  Port=4
  Theta : Inport  Port=5
  Psi : Inport  Port=6
  U1 : Inport  Port=7
  Constant : Constant  Value=m
  Divide : Product  Inputs=*/
  Subsystem : Subsystem
  Subsystem1 : Subsystem
  Subsystem2 : Subsystem
  X dot dot : Outport  VectorParamsAs1DForOutWhenUnconnected=off
  Ydot dot : Outport  Port=2  VectorParamsAs1DForOutWhenUnconnected=off
  Z dot dot : Outport  Port=3  VectorParamsAs1DForOutWhenUnconnected=off
  wires:
  Phi/1 -> Subsystem2/2(Phi), Subsystem1/2(Phi), Subsystem/2(Phi)
  U1/1 -> Divide/1
  Constant/1 -> Divide/2
  Divide/1 -> Subsystem/5(U1/M), Subsystem2/4(U1/m), Subsystem1/5(U1/M)
  Subsystem/1(X_dot_dot) -> X dot dot/1
  Subsystem1/1(Y_dot_dot) -> Ydot dot/1
  Subsystem2/1(Z_dot_dot) -> Z dot dot/1
  Theta/1 -> Subsystem2/3(Theta), Subsystem1/3(Theta), Subsystem/3(Theta)
  Psi/1 -> Subsystem1/4(Psi), Subsystem/4(Psi)
  X_dot/1 -> Subsystem/1(X_dot)
  Y_dot/1 -> Subsystem1/1(Y_dot)
  Z_dot/1 -> Subsystem2/1(Z_dot)

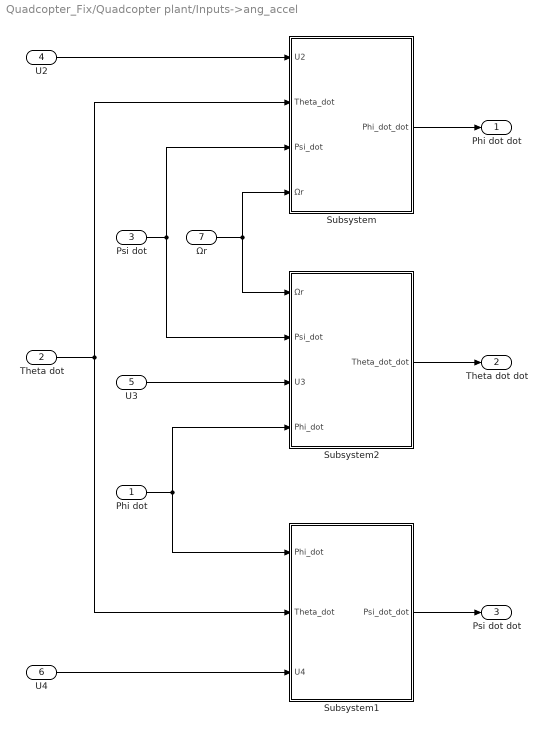
== system Quadcopter_Fix/Quadcopter plant/Inputs->ang_accel ==
  Phi dot : Inport
  Theta dot : Inport  Port=2
  Psi dot : Inport  Port=3
  U2 : Inport  Port=4
  U3 : Inport  Port=5
  U4 : Inport  Port=6
  Ωr : Inport  Port=7
  Subsystem : Subsystem
  Subsystem1 : Subsystem
  Subsystem2 : Subsystem
  Phi dot dot : Outport  VectorParamsAs1DForOutWhenUnconnected=off
  Theta dot dot : Outport  Port=2  VectorParamsAs1DForOutWhenUnconnected=off
  Psi dot dot : Outport  Port=3  VectorParamsAs1DForOutWhenUnconnected=off
  wires:
  U3/1 -> Subsystem2/3(U3)
  U4/1 -> Subsystem1/3(U4)
  Subsystem/1(Phi_dot_dot) -> Phi dot dot/1
  U2/1 -> Subsystem/1(U2)
  Ωr/1 -> Subsystem/4(Ωr), Subsystem2/1(Ωr)
  Psi dot/1 -> Subsystem2/2(Psi_dot), Subsystem/3(Psi_dot)
  Subsystem2/1(Theta_dot_dot) -> Theta dot dot/1
  Subsystem1/1(Psi_dot_dot) -> Psi dot dot/1
  Theta dot/1 -> Subsystem/2(Theta_dot), Subsystem1/2(Theta_dot)
  Phi dot/1 -> Subsystem2/4(Phi_dot), Subsystem1/1(Phi_dot)

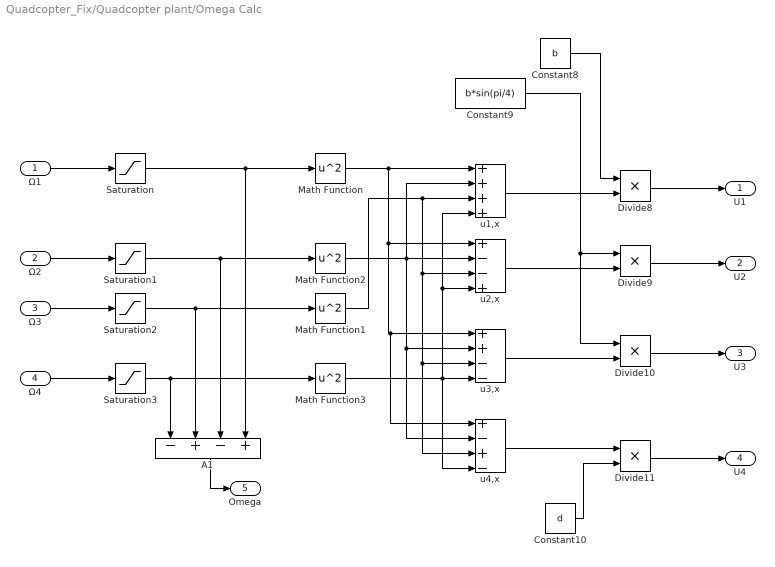
== system Quadcopter_Fix/Quadcopter plant/Omega Calc ==
  Ω1 : Inport
  Ω2 : Inport  Port=2
  Ω3 : Inport  Port=3
  Ω4 : Inport  Port=4
  A1 : Sum  Inputs=-+-+
  Constant10 : Constant  Value=d
  Constant8 : Constant  Value=b
  Constant9 : Constant  Value=b*sin(pi/4)
  Divide{8..11} (4 alike) : Product  Inputs=**
  Math Function{,1..3} (4 alike) : Math  Operator=square  SignedPower=on  SaturateOnIntegerOverflow=on
  Saturation{,1..3} (4 alike) : Saturate  UpperLimit=inf  LowerLimit=0
  u1,x : Sum  Inputs=++++
  u2,x : Sum  Inputs=+--+
  u3,x : Sum  Inputs=++--
  u4,x : Sum  Inputs=+-+-
  U1 : Outport  VectorParamsAs1DForOutWhenUnconnected=off
  U2 : Outport  Port=2  VectorParamsAs1DForOutWhenUnconnected=off
  U3 : Outport  Port=3  VectorParamsAs1DForOutWhenUnconnected=off
  U4 : Outport  Port=4  VectorParamsAs1DForOutWhenUnconnected=off
  Omega : Outport  Port=5  VectorParamsAs1DForOutWhenUnconnected=off
  wires:
  Constant10/1 -> Divide11/2
  u4,x/1 -> Divide11/1
  u3,x/1 -> Divide10/2
  u2,x/1 -> Divide9/2
  Constant9/1 -> Divide10/1, Divide9/1
  u1,x/1 -> Divide8/2
  Constant8/1 -> Divide8/1
  A1/1 -> Omega/1
  Divide8/1 -> U1/1
  Divide9/1 -> U2/1
  Divide10/1 -> U3/1
  Divide11/1 -> U4/1
  Math Function/1 -> u4,x/1, u3,x/1, u2,x/1, u1,x/1
  Math Function1/1 -> u4,x/3, u3,x/3, u2,x/3, u1,x/3
  Math Function2/1 -> u1,x/2, u4,x/2, u3,x/2, u2,x/2
  Math Function3/1 -> u1,x/4, u2,x/4, u4,x/4, u3,x/4
  Ω1/1 -> Saturation/1
  Ω2/1 -> Saturation1/1
  Ω3/1 -> Saturation2/1
  Ω4/1 -> Saturation3/1
  Saturation2/1 -> A1/2, Math Function1/1
  Saturation1/1 -> Math Function2/1, A1/3
  Saturation/1 -> Math Function/1, A1/4
  Saturation3/1 -> A1/1, Math Function3/1

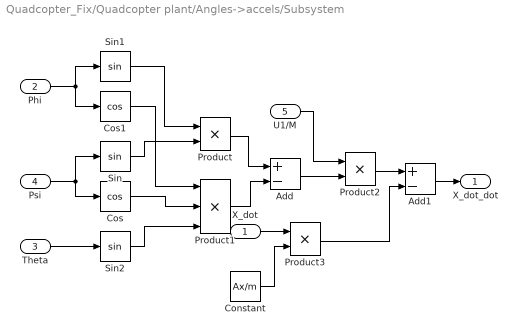
== system Quadcopter_Fix/Quadcopter plant/Angles->accels/Subsystem ==
  X_dot : Inport
  Phi : Inport  Port=2
  Theta : Inport  Port=3
  Psi : Inport  Port=4
  U1/M : Inport  Port=5
  Add : Sum  Inputs=+-
  Add1 : Sum  Inputs=+-
  Constant : Constant  Value=Ax/m
  Cos : Trigonometry  Operator=cos
  Cos1 : Trigonometry  Operator=cos
  Product : Product
  Product1 : Product  Inputs=3
  Product2 : Product
  Product3 : Product
  Sin : Trigonometry
  Sin1 : Trigonometry
  Sin2 : Trigonometry
  X_dot_dot : Outport  VectorParamsAs1DForOutWhenUnconnected=off
  wires:
  Product1/1 -> Add/2
  Product/1 -> Add/1
  U1/M/1 -> Product2/1
  Add/1 -> Product2/2
  Psi/1 -> Cos/1, Sin/1
  Phi/1 -> Cos1/1, Sin1/1
  Theta/1 -> Sin2/1
  Cos1/1 -> Product1/1
  Cos/1 -> Product1/2
  Sin2/1 -> Product1/3
  Sin1/1 -> Product/1
  Sin/1 -> Product/2
  Product2/1 -> Add1/1
  Add1/1 -> X_dot_dot/1
  X_dot/1 -> Product3/1
  Constant/1 -> Product3/2
  Product3/1 -> Add1/2

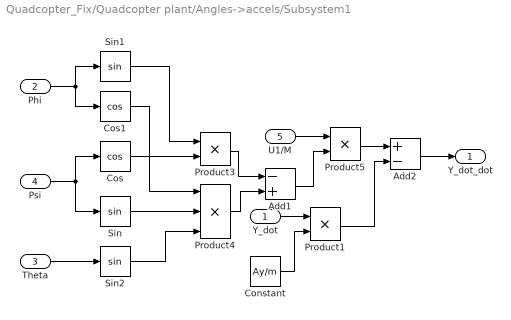
== system Quadcopter_Fix/Quadcopter plant/Angles->accels/Subsystem1 ==
  Y_dot : Inport
  Phi : Inport  Port=2
  Theta : Inport  Port=3
  Psi : Inport  Port=4
  U1/M : Inport  Port=5
  Add1 : Sum  Inputs=-+
  Add2 : Sum  Inputs=+-
  Constant : Constant  Value=Ay/m
  Cos : Trigonometry  Operator=cos
  Cos1 : Trigonometry  Operator=cos
  Product1 : Product
  Product3 : Product
  Product4 : Product  Inputs=3
  Product5 : Product
  Sin : Trigonometry
  Sin1 : Trigonometry
  Sin2 : Trigonometry
  Y_dot_dot : Outport  VectorParamsAs1DForOutWhenUnconnected=off
  wires:
  Psi/1 -> Sin/1, Cos/1
  Phi/1 -> Cos1/1, Sin1/1
  Theta/1 -> Sin2/1
  Add1/1 -> Product5/2
  Product4/1 -> Add1/2
  U1/M/1 -> Product5/1
  Product3/1 -> Add1/1
  Cos1/1 -> Product4/1
  Sin/1 -> Product4/2
  Sin2/1 -> Product4/3
  Sin1/1 -> Product3/1
  Cos/1 -> Product3/2
  Y_dot/1 -> Product1/1
  Constant/1 -> Product1/2
  Product1/1 -> Add2/2
  Product5/1 -> Add2/1
  Add2/1 -> Y_dot_dot/1

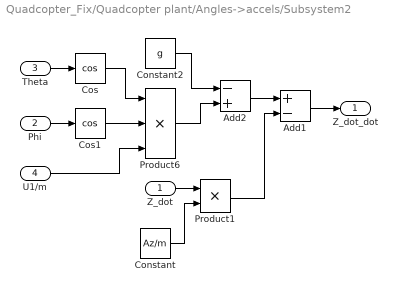
== system Quadcopter_Fix/Quadcopter plant/Angles->accels/Subsystem2 ==
  Z_dot : Inport
  Phi : Inport  Port=2
  Theta : Inport  Port=3
  U1/m : Inport  Port=4
  Add1 : Sum  Inputs=+-
  Add2 : Sum  Inputs=-+
  Constant : Constant  Value=Az/m
  Constant2 : Constant  Value=g
  Cos : Trigonometry  Operator=cos
  Cos1 : Trigonometry  Operator=cos
  Product1 : Product
  Product6 : Product  Inputs=3
  Z_dot_dot : Outport  VectorParamsAs1DForOutWhenUnconnected=off
  wires:
  Phi/1 -> Cos1/1
  Theta/1 -> Cos/1
  U1/m/1 -> Product6/3
  Constant2/1 -> Add2/1
  Cos/1 -> Product6/1
  Product6/1 -> Add2/2
  Cos1/1 -> Product6/2
  Product1/1 -> Add1/2
  Z_dot/1 -> Product1/1
  Constant/1 -> Product1/2
  Add2/1 -> Add1/1
  Add1/1 -> Z_dot_dot/1

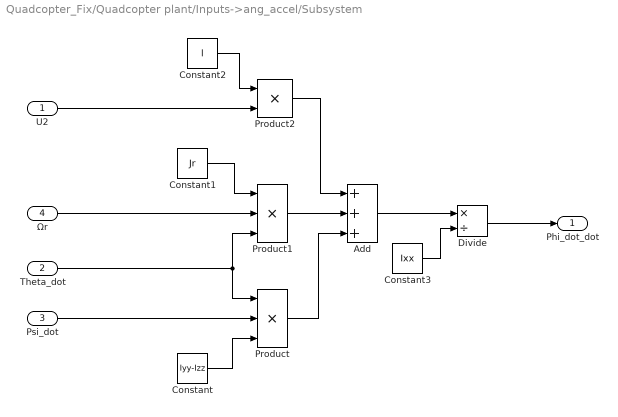
== system Quadcopter_Fix/Quadcopter plant/Inputs->ang_accel/Subsystem ==
  U2 : Inport
  Theta_dot : Inport  Port=2
  Psi_dot : Inport  Port=3
  Ωr : Inport  Port=4
  Add : Sum  Inputs=+++
  Constant : Constant  Value=Iyy-Izz
  Constant1 : Constant  Value=Jr
  Constant2 : Constant  Value=l
  Constant3 : Constant  Value=Ixx
  Divide : Product  Inputs=*/
  Product : Product  Inputs=3
  Product1 : Product  Inputs=3
  Product2 : Product
  Phi_dot_dot : Outport  VectorParamsAs1DForOutWhenUnconnected=off
  wires:
  Psi_dot/1 -> Product/2
  Theta_dot/1 -> Product/1, Product1/3
  Constant/1 -> Product/3
  Ωr/1 -> Product1/2
  Constant1/1 -> Product1/1
  U2/1 -> Product2/2
  Constant2/1 -> Product2/1
  Product1/1 -> Add/2
  Product2/1 -> Add/1
  Product/1 -> Add/3
  Add/1 -> Divide/1
  Constant3/1 -> Divide/2
  Divide/1 -> Phi_dot_dot/1

== system Quadcopter_Fix/Quadcopter plant/Inputs->ang_accel/Subsystem1 ==
  Phi_dot : Inport
  Theta_dot : Inport  Port=2
  U4 : Inport  Port=3
  Add2 : Sum
  Constant11 : Constant  Value=Izz
  Constant8 : Constant  Value=Ixx-Iyy
  Divide2 : Product  Inputs=*/
  Product6 : Product  Inputs=3
  Psi_dot_dot : Outport  VectorParamsAs1DForOutWhenUnconnected=off
  wires:
  Theta_dot/1 -> Product6/1
  Phi_dot/1 -> Product6/2
  Constant8/1 -> Product6/3
  Add2/1 -> Divide2/1
  Constant11/1 -> Divide2/2
  Divide2/1 -> Psi_dot_dot/1
  Product6/1 -> Add2/2
  U4/1 -> Add2/1

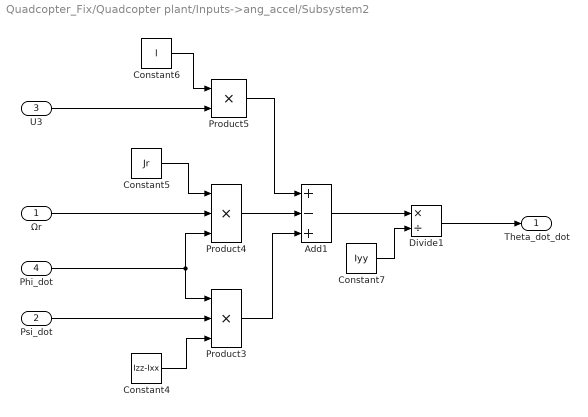
== system Quadcopter_Fix/Quadcopter plant/Inputs->ang_accel/Subsystem2 ==
  Ωr : Inport
  Psi_dot : Inport  Port=2
  U3 : Inport  Port=3
  Phi_dot : Inport  Port=4
  Add1 : Sum  Inputs=+-+
  Constant4 : Constant  Value=Izz-Ixx
  Constant5 : Constant  Value=Jr
  Constant6 : Constant  Value=l
  Constant7 : Constant  Value=Iyy
  Divide1 : Product  Inputs=*/
  Product3 : Product  Inputs=3
  Product4 : Product  Inputs=3
  Product5 : Product
  Theta_dot_dot : Outport  VectorParamsAs1DForOutWhenUnconnected=off
  wires:
  Psi_dot/1 -> Product3/2
  Phi_dot/1 -> Product3/1, Product4/3
  Ωr/1 -> Product4/2
  Constant4/1 -> Product3/3
  Constant5/1 -> Product4/1
  U3/1 -> Product5/2
  Constant6/1 -> Product5/1
  Product4/1 -> Add1/2
  Product5/1 -> Add1/1
  Product3/1 -> Add1/3
  Add1/1 -> Divide1/1
  Constant7/1 -> Divide1/2
  Divide1/1 -> Theta_dot_dot/1

== matlab function Quadcopter_Fix/Embedded MATLAB Function ==
  settings: fimath=|
      | fimath(...
      | 'RoundMode', 'floor',...
      | 'OverflowMode', 'wrap',...
      | 'ProductMode', 'KeepLSB', 'ProductWordLength', 32,...
      | 'SumMode', 'KeepLSB', 'SumWordLength', 32,...
      | 'CastBeforeSum', false)
  data: u input; axisangle output
function axisangle = fcn(u)
% This block supports an embeddable subset of the MATLAB language.
% See the help menu for details.

heading = u(3); % yaw
attitude = u(2); % pitch
bank = u(1); % roll

c1 = cos(heading/2);
s1 = sin(heading/2);
c2 = cos(attitude/2);
s2 = sin(attitude/2);
c3 = cos(bank/2);
s3 = sin(bank/2);
% c1c2 = c1*c2;
% s1s2 = s1*s2;
w =c1*c2*c3 - s1*s2*s3;
x =c1*c2*s3 + s1*s2*c3;
y =s1*c2*c3 + c1*s2*s3;
z =c1*s2*c3 - s1*c2*s3;
angle = 2 * acos(w);
norm = x*x+y*y+z*z;
if (norm < 0.001) % when all euler angles are zero angle =0 so we can set axis to anything to avoid divide by zero
    x=1;
    y=0;
    z=0;
else
    norm = sqrt(norm);
    x =x/ norm;
    y =y/ norm;
    z =z/ norm;
end
axisangle = [x y z angle];
